simulink model "Exercitiul3"  (R2016a)
settings: Solver=VariableStepDiscrete  StartTime=0.0  StopTime=2400  RelTol=1e-3
undefined symbols (not defined in the file): m, n
settings Model: Creator=Cristina  LastModifiedBy=Cristina

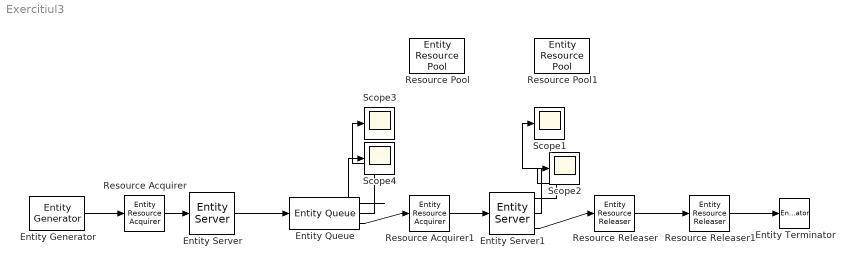
== system Exercitiul3 ==
  Entity Generator : EntityGenerator  OutputPortMessageModes=m  TimeSource=MATLAB action  IntergenerationTimeAction=|  EntityType=Structured  EntityTypeName=Entity
      | persistent count
      | if(isempty(count))
      |     count = 1;
      | end
      | if(count < 5)
      |     dt = 0;
      |     count = count + 1;
      | else
      |     dt = inf;
      | end
  Entity Queue : EntityQueue  InputPortMessageModes=m  OutputPortMessageModes=n,n,m  NumberEntitiesInBlock=on  AverageWait=on
      settings: OutputPortMap=o1,o2,o5
  Entity Server : EntityServer  InputPortMessageModes=m  OutputPortMessageModes=m  Capacity=4  ServiceTimeSource=MATLAB action  ServiceTimeAction=dt = 25 + rand * 10;
  Entity Server1 : EntityServer  InputPortMessageModes=m  OutputPortMessageModes=n,n,m  Capacity=1  ServiceTimeSource=MATLAB action  ServiceTimeAction=dt = 6 + rand * 4;  AverageWait=on  Utilization=on
      settings: OutputPortMap=o4,o5,o9
  Entity Terminator : EntityTerminator  InputPortMessageModes=m
  Resource Acquirer : EntityResourceAcquirer  InputPortMessageModes=m  OutputPortMessageModes=m  NumberWaitingEntities=5  ResourceName=Muncitori
      settings: OutputPortMap=o3
  Resource Acquirer1 : EntityResourceAcquirer  InputPortMessageModes=m  OutputPortMessageModes=m  NumberWaitingEntities=5  ResourceName=Cuptor
      settings: OutputPortMap=o3
  Resource Releaser : EntityResourceReleaser  InputPortMessageModes=m  OutputPortMessageModes=m  ResourceToRelease=Selected  ResourceName=Cuptor
  Resource Releaser1 : EntityResourceReleaser  InputPortMessageModes=m  OutputPortMessageModes=m  ResourceToRelease=Selected  ResourceName=Muncitori
  Resource Pool : EntityResourcePool  ResourceName=Muncitori  ResourceAmount=4
  Resource Pool1 : EntityResourcePool  ResourceName=Cuptor  ResourceAmount=1
  Scope{1..4} (4 alike) : Scope
  wires:
  Resource Acquirer1/1 -> Entity Server1/1
  Entity Generator/1 -> Resource Acquirer/1
  Resource Acquirer/1 -> Entity Server/1
  Entity Server/1 -> Entity Queue/1
  Entity Server1/3 -> Resource Releaser/1
  Resource Releaser/1 -> Resource Releaser1/1
  Entity Server1/1 -> Scope2/1
  Resource Releaser1/1 -> Entity Terminator/1
  Entity Server1/2 -> Scope1/1
  Entity Queue/3 -> Resource Acquirer1/1
  Entity Queue/2 -> Scope3/1
  Entity Queue/1 -> Scope4/1
